simulink model "intentRecBle"  (R2020a)
settings: Solver=FixedStepAuto  StartTime=0.0  StopTime=10.0  RelTol=1e-3
undefined symbols (not defined in the file): blue, blue2, blue3, green, green2, green3, red, red2, red3
libraries: simulink x4, androidaudiovideolib x3, androiduilib x3, androidcommunicationlib x2
settings Model: Creator=luisi  LastModifiedBy=luisi
settings OptimizationCC: EnhancedBackFolding=on  PassReuseOutputArgsAs=Individual arguments  ZeroExternalMemoryAtStartup=off  ZeroInternalMemoryAtStartup=off  MaxStackSize=64  OptimizeBlockOrder=speed  DifferentSizesBufferReuse=on  OptimizationCustomize=off  EfficientTunableParamExpr=on
settings DebuggingCC: ParameterTunabilityLossMsg=error
settings HardwareCC: ProdBitPerPointer=32  ProdBitPerSizeT=32  ProdBitPerPtrDiffT=32  ProdLargestAtomicInteger=Long  ProdLargestAtomicFloat=Double  ProdWordSize=32  ProdHWDeviceType=ARM Compatible->ARM Cortex
settings SFSimCC: MATLABDynamicMemAlloc=off
settings RTWCC: SystemTargetFile=ert.tlc  HardwareBoard=Android Device  TemplateMakefile=ert_default_tmf  RTWVerbose=off  Toolchain=Android SDK/NDK Tools
settings CodeAppCC: ForceParamTrailComments=on  IgnoreCustomStorageClasses=off  OperatorAnnotations=on  SimulinkDataObjDesc=on  SFDataObjDesc=on  InsertBlockDesc=on

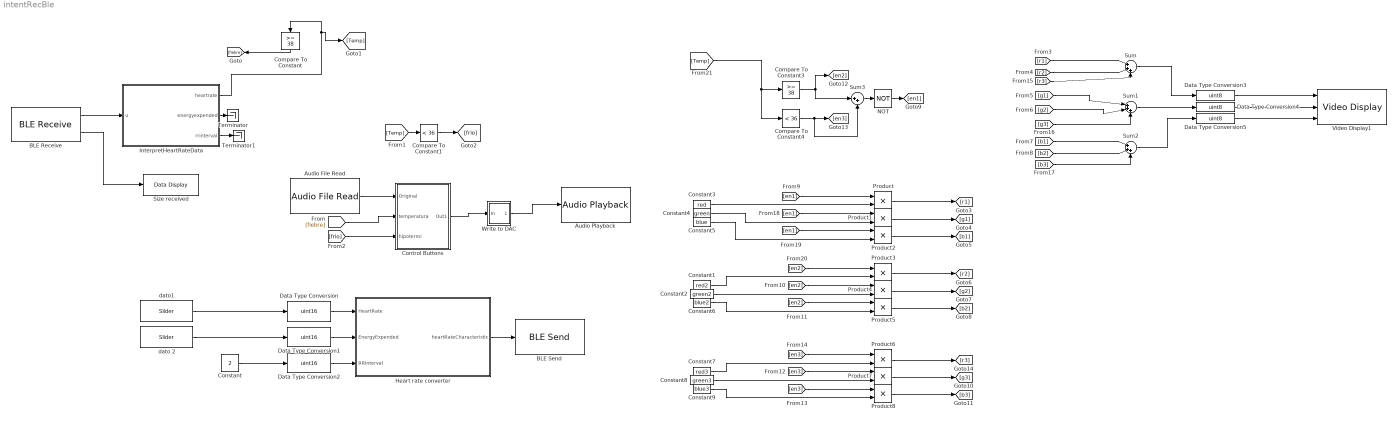
== system intentRecBle ==
  Audio File Read : androidaudiovideolib/Audio File Read  FileName=C:\Users\luisi\Downloads\baby.mp3  FrameSize=4410
      settings: SourceProductBaseCode=ANDROID
  Audio Playback : androidaudiovideolib/Audio Playback  SampleFreq=44100  AudioSamplingFreq=44100  SampleTime=0.1  DeviceStr=0  QueueDuration=0  BlockPlatform=Android
      settings: SourceProductBaseCode=ANDROID
  BLE Receive : androidcommunicationlib/BLE Receive  DeviceMode=Central (Client)  BluetoothAddress=43:33:83:91:21:94  CharUUID=00002a37-0000-1000-8000-00805f9b34fb  ServiceUUID=0000180d-0000-1000-8000-00805f9b34fb  device=RedmiLuisa  character="Heart Rate\\Heart Rate  Measurement"  CustomService=off  ServiceName=Heart Rate  CharacteristicName="Heart Rate  Measurement"  CustomServiceUUID=<Enter Service UUID>  CustomCharUUID=<Enter Characteristic UUID>  DataSize=7  SampleTime=0.1  charseruuid=00001801-0000-1000-8000-00805f9b34fb\00002a05-0000-1000-8000-00805f9b34fb  seruuid=00001810-0000-1000-8000-00805f9b34fb  PeripheralService=0000180d-0000-1000-8000-00805f9b34fb  PeripheralCharacteristic=00002a37-0000-1000-8000-00805f9b34fb  chruuid=00002a37-0000-1000-8000-00805f9b34fb  BLEId=intentRecBle/BLE_Receive  Devicename=RedmiLuisa  IsCustomService=0
      settings: SourceProductBaseCode=ANDROID
  BLE Send : androidcommunicationlib/BLE Send  DeviceMode=Peripheral (Server)  BluetoothAddress=43:33:83:91:21:94  CharUUID=00002a05-0000-1000-8000-00805f9b34fb  ServiceUUID=00001801-0000-1000-8000-00805f9b34fb  device=RedmiLuisa  character=Generic Attribute\Service Changed  CustomService=off  ServiceName=Heart Rate  CharacteristicName="Heart Rate  Measurement"  CustomServiceUUID=<Enter Service UUID>  CustomCharUUID=<Enter Characteristic UUID>  charseruuid=00001801-0000-1000-8000-00805f9b34fb\00002a05-0000-1000-8000-00805f9b34fb  seruuid=00001810-0000-1000-8000-00805f9b34fb  chruuid=00002a37-0000-1000-8000-00805f9b34fb  PeripheralService=0000180d-0000-1000-8000-00805f9b34fb  PeripheralCharacteristic=00002a37-0000-1000-8000-00805f9b34fb  BLEId=intentRecBle/BLE_Send  Devicename=RedmiLuisa  IsCustomService=0  Size=-1
      settings: SourceProductBaseCode=ANDROID
  Compare To Constant : simulink/Logic and Bit Operations/Compare To Constant  relop=>=  const=38  OutDataTypeStr=boolean
  Compare To Constant1 : simulink/Logic and Bit Operations/Compare To Constant  relop=<  const=36  OutDataTypeStr=boolean
  Compare To Constant3 : simulink/Logic and Bit Operations/Compare To Constant  relop=>=  const=38  OutDataTypeStr=uint8
  Compare To Constant4 : simulink/Logic and Bit Operations/Compare To Constant  relop=<  const=36  OutDataTypeStr=uint8
  Constant : Constant  Value=2
  Constant1 : Constant  Value=red2
  Constant2 : Constant  Value=green2
  Constant3 : Constant  Value=red
  Constant4 : Constant  Value=green
  Constant5 : Constant  Value=blue
  Constant6 : Constant  Value=blue2
  Constant7 : Constant  Value=red3
  Constant8 : Constant  Value=green3
  Constant9 : Constant  Value=blue3
  Control Buttons : Subsystem
  Data Type Conversion : DataTypeConversion  OutDataTypeStr=uint16
  Data Type Conversion1 : DataTypeConversion  OutDataTypeStr=uint16
  Data Type Conversion2 : DataTypeConversion  OutDataTypeStr=uint16
  Data Type Conversion3 : DataTypeConversion  OutDataTypeStr=uint8
  Data Type Conversion4 : DataTypeConversion  OutDataTypeStr=uint8
  Data Type Conversion5 : DataTypeConversion  OutDataTypeStr=uint8
  Heart rate converter : MATLAB Function  TreatAsAtomicUnit=on
  InterpretHeartRateData : MATLAB Function  TreatAsAtomicUnit=on
  NOT : Logic  Operator=NOT  IconShape=distinctive  AllPortsSameDT=off  OutDataTypeStr=boolean
  Product{,1..8} (9 alike) : Product
  Size received : androiduilib/Data Display  DataDisplayId=intentRecBle/Size_received  Format=Float  Precision=6  SimulateUsing=Code generation  blockPlatform=Android
      settings: SourceProductBaseCode=ANDROID
  Sum : Sum  Inputs=|+++
  Sum1 : Sum  Inputs=|+++
  Sum2 : Sum  Inputs=|+++
  Sum3 : Sum  Inputs=|++
  Terminator : Terminator
  Terminator1 : Terminator
  Video Display1 : androidaudiovideolib/Video Display  BlockPlatform=Android
      settings: SourceProductBaseCode=ANDROID
  Write to DAC : Subsystem
  dato 2 : androiduilib/Slider  Min=0  Value=0  Max=5  Resolution=1  SliderId=intentRecBle/dato_2  SampleTime=0.1  BlockPlatform=Android
      settings: SourceProductBaseCode=ANDROID
  dato1 : androiduilib/Slider  Min=0  Value=0  Max=5  Resolution=1  SliderId=intentRecBle/dato1  SampleTime=0.1  BlockPlatform=Android
      settings: SourceProductBaseCode=ANDROID
  wires:
  BLE Receive/2 -> Size received/1
  BLE Receive/1 -> InterpretHeartRateData/1(u)
  Data Type Conversion2/1 -> Heart rate converter/3(RRInterval)
  Data Type Conversion1/1 -> Heart rate converter/2(EnergyExpended)
  Heart rate converter/1(heartRateCharacteristic) -> BLE Send/1
  Data Type Conversion/1 -> Heart rate converter/1(HeartRate)
  Compare To Constant/1 -> [fiebre]
  Audio File Read/1 -> Control Buttons/1(Original)
  InterpretHeartRateData/1(heartrate) -> [Temp], Compare To Constant/1
  [frio] -> Control Buttons/3(hipotermi)
  Write to DAC/1(Out) -> Audio Playback/1
  [Temp] -> Compare To Constant1/1
  Control Buttons/1(Out1) -> Write to DAC/1(In)
  Compare To Constant1/1 -> [frio]
  [fiebre] -> Control Buttons/2(temperatura)
  InterpretHeartRateData/2(energyexpended) -> Terminator/1
  InterpretHeartRateData/3(rrinterval) -> Terminator1/1
  dato1/1 -> Data Type Conversion/1
  dato 2/1 -> Data Type Conversion1/1
  Constant/1 -> Data Type Conversion2/1
  [b3] -> Sum2/3
  [g3] -> Sum1/3
  Constant1/1 -> Product3/2
  Constant7/1 -> Product6/2
  Sum/1 -> Data Type Conversion3/1
  Data Type Conversion5/1 -> Video Display1/3
  [Temp] -> Compare To Constant4/1, Compare To Constant3/1
  [en3] -> Product8/1
  Constant8/1 -> Product7/2
  [en3] -> Product6/1
  Product1/1 -> [g1]
  Sum2/1 -> Data Type Conversion5/1
  [r3] -> Sum/3
  Product6/1 -> [r3]
  Product7/1 -> [g3]
  [en2] -> Product5/1
  [en3] -> Product7/1
  [en2] -> Product3/1
  Compare To Constant3/1 -> Sum3/1, [en2]
  [en2] -> Product4/1
  Data Type Conversion3/1 -> Video Display1/1
  [g1] -> Sum1/1
  Product4/1 -> [g2]
  [r2] -> Sum/2
  Product/1 -> [r1]
  Product3/1 -> [r2]
  [b2] -> Sum2/2
  Constant3/1 -> Product/2
  Sum1/1 -> Data Type Conversion4/1
  Compare To Constant4/1 -> [en3], Sum3/2
  Constant6/1 -> Product5/2
  [en1] -> Product2/1
  [g2] -> Sum1/2
  [en1] -> Product/1
  Constant2/1 -> Product4/2
  Product5/1 -> [b2]
  [r1] -> Sum/1
  Constant9/1 -> Product8/2
  Constant4/1 -> Product1/2
  Constant5/1 -> Product2/2
  Product2/1 -> [b1]
  Data Type Conversion4/1 -> Video Display1/2
  [b1] -> Sum2/1
  Product8/1 -> [b3]
  [en1] -> Product1/1
  NOT/1 -> [en1]
  Sum3/1 -> NOT/1

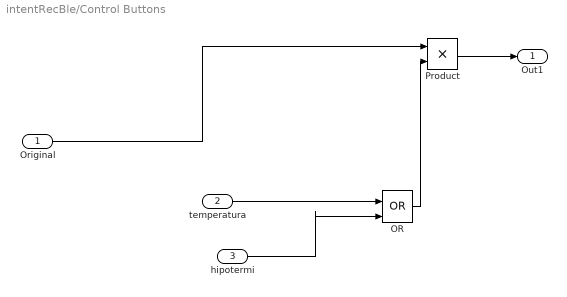
== system intentRecBle/Control Buttons ==
  Original : Inport
  temperatura : Inport  Port=2
  hipotermi : Inport  Port=3
  OR : Logic  Operator=OR  IconShape=distinctive  AllPortsSameDT=off  OutDataTypeStr=boolean
  Product : Product
  Out1 : Outport  VectorParamsAs1DForOutWhenUnconnected=off
  wires:
  Product/1 -> Out1/1
  Original/1 -> Product/1
  temperatura/1 -> OR/1
  hipotermi/1 -> OR/2
  OR/1 -> Product/2

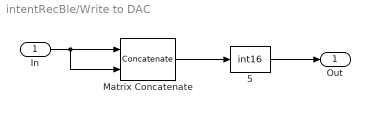
== system intentRecBle/Write to DAC ==
  In : Inport
  " 5" : DataTypeConversion  OutDataTypeStr=int16
  Matrix Concatenate : Concatenate  Mode=Multidimensional array  ConcatenateDimension=2
  Out : Outport  VectorParamsAs1DForOutWhenUnconnected=off
  wires:
  In/1 -> Matrix Concatenate/2, Matrix Concatenate/1
  Matrix Concatenate/1 -> " 5"/1
  " 5"/1 -> Out/1

== matlab function intentRecBle/Heart rate converter ==
  data: HeartRate input; heartRateCharacteristic output; EnergyExpended input; RRInterval input
function heartRateCharacteristic = ConvertToHeartRateFormat(HeartRate, EnergyExpended, RRInterval)
flag = uint8(25);
heartRateCharacteristic = zeros(7,1,'uint8');
heartRateCharacteristic(1)= flag;
[lower, upper] = getBytes(HeartRate);
heartRateCharacteristic(2) = lower;
heartRateCharacteristic(3) = upper;
[lower, upper] = getBytes(EnergyExpended);
heartRateCharacteristic(4) = lower;
heartRateCharacteristic(5) = upper;
[lower, upper] = getBytes(RRInterval);
heartRateCharacteristic(6) = lower;
heartRateCharacteristic(7) = upper;
end

function [lower,upper] = getBytes(parameter)
h = dec2bin(parameter,16);
lower = bin2dec(h(9:16));
upper= bin2dec(h(1:8));
end

== matlab function intentRecBle/InterpretHeartRateData ==
  data: u input; heartrate output; energyexpended output; rrinterval output
function [heartrate, energyexpended, rrinterval ] = InterpretHeartRateData(u)
flag = uint8(u(1));
heartrate = uint16(0);
energyexpended=uint16(0);
rrinterval = uint16(0);
b = bitget(flag,8:-1:1);

 if b(8) == 0
     format = uint8(2);
     heartrate = uint16(u(2));
 else
     format = uint8(3);
     heartrate = typecast([u(2) u(3)], 'uint16');
 end
 
 if b(5) == 1
     energy = uint8(2);
     energyexpended = typecast([u(format +1) u(format + 2)], 'uint16');
 else
     energy = uint8(0);
     energyexpended = uint16(0);
 end
 
 if b(4) == 1
     rrinterval = typecast([u(format +energy + 1) u(format + energy + 2)],'uint16');
 else
     rrinterval = uint16(0);
 end
end
